simulink model "sampleModel248"  (R2021b)
settings: Solver=VariableStepAuto  StartTime=0.0  StopTime=10.0  RelTol=1e-3
undefined symbols (not defined in the file or in its folder): Newton, Raphson
libraries: simulink x15, slpidlib x4
settings Model: Creator=user  LastModifiedBy=user

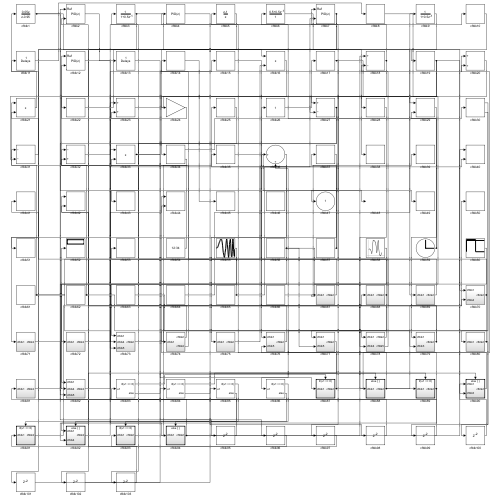
[thumbnail: Simulink's stored preview of the top-level diagram]
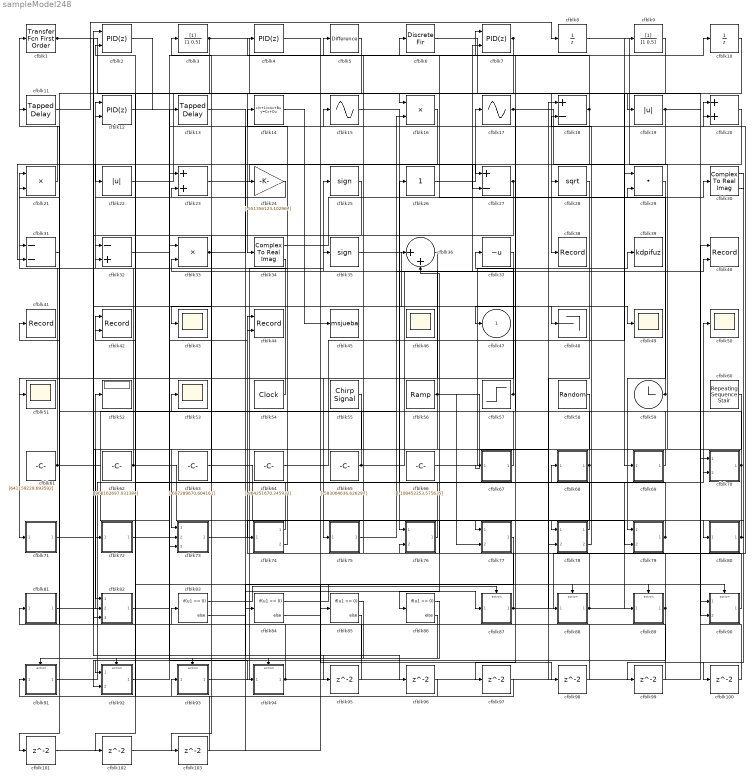
== system sampleModel248 ==
  cfblk1 : simulink/Discrete/Transfer Fcn First Order  PoleZ=0.95  ICPrevOutput=0.0  DoSatur=off
  cfblk10 : UnitDelay  HasFrameUpgradeWarning=on
  cfblk{95..103} (9 alike) : Delay  SampleTime=1
  cfblk11 : simulink/Discrete/Tapped Delay  vinit=0.0  samptime=-1  NumDelays=1  DelayOrder=Oldest  includeCurrent=off
  cfblk12 : slpidlib/PID Controller (2DOF)  Controller=PID  Form=Parallel  TimeDomain=Discrete-time  UseExternalTs=off  SampleTime=1  IntegratorMethod=Forward Euler  FilterMethod=Forward Euler  ControllerParametersSource=internal  P=1  I=1  D=0  UseFilter=on  N=100  b=1  c=1  TunerSelectOption=Transfer Function Based (PID Tuner App)  InitialConditionSource=internal  InitialConditionForIntegrator=0  InitialConditionForFilter=0  DifferentiatorICPrevScaledInput=0  ExternalReset=none  TrackingMode=off  Kt=1  LimitOutput=off  SatLimitsSource=internal  UpperSaturationLimit=inf  LowerSaturationLimit=-inf  LinearizeAsGain=off  AntiWindupMode=none  Kb=1  POutMin=[]  POutMax=[]  IOutMin=[]  IOutMax=[]  DOutMin=[]  DOutMax=[]  NOutMin=[]  NOutMax=[]  bOutMin=[]  bOutMax=[]  cOutMin=[]  cOutMax=[]  SumOutMin=[]  SumOutMax=[]  SaturationOutMin=[]  SaturationOutMax=[]  PParamMin=[]  PParamMax=[]  IParamMin=[]  IParamMax=[]  DParamMin=[]  DParamMax=[]  NParamMin=[]  NParamMax=[]  bParamMin=[]  bParamMax=[]  cParamMin=[]  cParamMax=[]  KbParamMin=[]  KbParamMax=[]  KtParamMin=[]  KtParamMax=[]  KbOutMin=[]  KbOutMax=[]  KtOutMin=[]  KtOutMax=[]  IntegratorOutMin=[]  IntegratorOutMax=[]  FilterOutMin=[]  FilterOutMax=[]  SumI1OutMin=[]  SumI1OutMax=[]  SumI2OutMin=[]  SumI2OutMax=[]  SumI3OutMin=[]  SumI3OutMax=[]  SumI4OutMin=[]  SumI4OutMax=[]  SumDOutMin=[]  SumDOutMax=[]  Sum1OutMin=[]  Sum1OutMax=[]  Sum2OutMin=[]  Sum2OutMax=[]  Sum3OutMin=[]  Sum3OutMax=[]  DifferentiatorOutMin=[]  DifferentiatorOutMax=[]  FilterDiffOutCoefMin=[]  FilterDiffOutCoefMax=[]  ReciprocalOutMin=[]  ReciprocalOutMax=[]  SumDenOutMin=[]  SumDenOutMax=[]  SumNumOutMin=[]  SumNumOutMax=[]  DivideOutMin=[]  DivideOutMax=[]  UdiffTsProdOutMin=[]  UdiffTsProdOutMax=[]  NTsProdOutMin=[]  NTsProdOutMax=[]  UintegralTsProdOutMin=[]  UintegralTsProdOutMax=[]  UngainTsProdOutMin=[]  UngainTsProdOutMax=[]  IntegratorContinuousStateAttributes=''  IntegratorStateMustResolveToSignalObject=off  IntegratorRTWStateStorageClass=Auto  FilterContinuousStateAttributes=''  FilterStateMustResolveToSignalObject=off  FilterRTWStateStorageClass=Auto  ParallelPVariant=InternalParameters  IdealPVariant=Disabled  IVariant=InternalParameters  DVariant=InternalParameters  bVariant=InternalParameters  cVariant=InternalParameters  IntegratorVariant=Discrete  SatVariant=Disabled  AWVariant=Passthrough  PCopyVariant=Disabled  TRVariant=Disabled  FdbkBlocksVariant=Forward  IdealPFdbkVariant=Disabled  SatFdbkVariant=Disabled  DerivativeFilterVariant=ForwardEulerFilter  NVariant=InternalParameters  NCopyVariant=Disabled  FilterICVariant=InternalICsFilter  IntegratorICVariant=InternalICs  ExternalResetVariant=Disabled  TRSumVariant=Passthrough  SumFdbkVariant=Disabled  SumVariant=Sum_PID  TsampFilterVariant=InternalTs  TsampNgainVariant=Passthrough  TsampIntegralVariant=Passthrough  ExternalSaturationOutDataTypeStr=Inherit: Same as second input
      settings: SourceProductBaseCode=SL
  cfblk13 : simulink/Discrete/Tapped Delay  vinit=0.0  samptime=-1  NumDelays=1  DelayOrder=Oldest  includeCurrent=off
  cfblk14 : DiscreteStateSpace
  cfblk15 : Sin  TimeSource=Use external signal  SampleTime=0
  cfblk16 : Product  Inputs=**
  cfblk17 : Sin  TimeSource=Use external signal  SampleTime=0
  cfblk18 : Sum  Inputs=+-
  cfblk19 : Abs
  cfblk2 : slpidlib/PID Controller (2DOF)  Controller=PID  Form=Parallel  TimeDomain=Discrete-time  UseExternalTs=off  SampleTime=1  IntegratorMethod=Forward Euler  FilterMethod=Forward Euler  ControllerParametersSource=internal  P=1  I=1  D=0  UseFilter=on  N=100  b=1  c=1  TunerSelectOption=Transfer Function Based (PID Tuner App)  InitialConditionSource=internal  InitialConditionForIntegrator=0  InitialConditionForFilter=0  DifferentiatorICPrevScaledInput=0  ExternalReset=none  TrackingMode=off  Kt=1  LimitOutput=off  SatLimitsSource=internal  UpperSaturationLimit=inf  LowerSaturationLimit=-inf  LinearizeAsGain=off  AntiWindupMode=none  Kb=1  POutMin=[]  POutMax=[]  IOutMin=[]  IOutMax=[]  DOutMin=[]  DOutMax=[]  NOutMin=[]  NOutMax=[]  bOutMin=[]  bOutMax=[]  cOutMin=[]  cOutMax=[]  SumOutMin=[]  SumOutMax=[]  SaturationOutMin=[]  SaturationOutMax=[]  PParamMin=[]  PParamMax=[]  IParamMin=[]  IParamMax=[]  DParamMin=[]  DParamMax=[]  NParamMin=[]  NParamMax=[]  bParamMin=[]  bParamMax=[]  cParamMin=[]  cParamMax=[]  KbParamMin=[]  KbParamMax=[]  KtParamMin=[]  KtParamMax=[]  KbOutMin=[]  KbOutMax=[]  KtOutMin=[]  KtOutMax=[]  IntegratorOutMin=[]  IntegratorOutMax=[]  FilterOutMin=[]  FilterOutMax=[]  SumI1OutMin=[]  SumI1OutMax=[]  SumI2OutMin=[]  SumI2OutMax=[]  SumI3OutMin=[]  SumI3OutMax=[]  SumI4OutMin=[]  SumI4OutMax=[]  SumDOutMin=[]  SumDOutMax=[]  Sum1OutMin=[]  Sum1OutMax=[]  Sum2OutMin=[]  Sum2OutMax=[]  Sum3OutMin=[]  Sum3OutMax=[]  DifferentiatorOutMin=[]  DifferentiatorOutMax=[]  FilterDiffOutCoefMin=[]  FilterDiffOutCoefMax=[]  ReciprocalOutMin=[]  ReciprocalOutMax=[]  SumDenOutMin=[]  SumDenOutMax=[]  SumNumOutMin=[]  SumNumOutMax=[]  DivideOutMin=[]  DivideOutMax=[]  UdiffTsProdOutMin=[]  UdiffTsProdOutMax=[]  NTsProdOutMin=[]  NTsProdOutMax=[]  UintegralTsProdOutMin=[]  UintegralTsProdOutMax=[]  UngainTsProdOutMin=[]  UngainTsProdOutMax=[]  IntegratorContinuousStateAttributes=''  IntegratorStateMustResolveToSignalObject=off  IntegratorRTWStateStorageClass=Auto  FilterContinuousStateAttributes=''  FilterStateMustResolveToSignalObject=off  FilterRTWStateStorageClass=Auto  ParallelPVariant=InternalParameters  IdealPVariant=Disabled  IVariant=InternalParameters  DVariant=InternalParameters  bVariant=InternalParameters  cVariant=InternalParameters  IntegratorVariant=Discrete  SatVariant=Disabled  AWVariant=Passthrough  PCopyVariant=Disabled  TRVariant=Disabled  FdbkBlocksVariant=Forward  IdealPFdbkVariant=Disabled  SatFdbkVariant=Disabled  DerivativeFilterVariant=ForwardEulerFilter  NVariant=InternalParameters  NCopyVariant=Disabled  FilterICVariant=InternalICsFilter  IntegratorICVariant=InternalICs  ExternalResetVariant=Disabled  TRSumVariant=Passthrough  SumFdbkVariant=Disabled  SumVariant=Sum_PID  TsampFilterVariant=InternalTs  TsampNgainVariant=Passthrough  TsampIntegralVariant=Passthrough  ExternalSaturationOutDataTypeStr=Inherit: Same as second input
      settings: SourceProductBaseCode=SL
  cfblk20 : Sum
  cfblk21 : Product
  cfblk22 : Abs
  cfblk23 : Sum
  cfblk24 : Gain  Gain=[-551356123.102967]
  cfblk25 : Signum
  cfblk26 : simulink/Math Operations/Slider Gain  gain=1  low=0  high=2
  cfblk27 : Sum  Inputs=+-
  cfblk28 : Sqrt  SaturateOnIntegerOverflow=on
  cfblk29 : DotProduct  InputSameDT=on  OutDataTypeStr=Inherit: Inherit via internal rule
  cfblk3 : DiscreteFilter  SampleTime=1
  cfblk30 : ComplexToRealImag
  cfblk31 : Sum  Inputs=--
  cfblk32 : Sum  Inputs=-+
  cfblk33 : Product  Inputs=**
  cfblk34 : ComplexToRealImag
  cfblk35 : Signum
  cfblk36 : Sum  Inputs=|++
  cfblk37 : UnaryMinus
  cfblk38 : Record  FileSettingsInternal="{\"entries\":[{\"content\":{\"excelSettings\":{\"content\":{},\"type\":\"Streamout.ExcelSettings\"}},\"type\":\"Streamout.FileSettingStorage\",\"uuid\":\"4657b973-2eff-446c-9fb0-9f6287b31807\"}],\"packageUris\":[\"http://schema.mathworks.com/mf0/streamout_blocks/R2020a\"],\"version\":\"1.0\"}"  SignalsInternal="{\"entries\":[{\"content\":{\"signals\":[{\"content\":{\"blockPath\":[\"sampleModel248/cfblk38\"],\"channel\":[],\"dimensions\":[1],\"domain\":\"sampleModel248/cfblk38\",\"lineColor\":\"#ff13a6\",\"plots\":[1],\"port\":1,\"sid\":[\"\"],\"signalID\":9988,\"signalName\":\"cfblk1\"},\"type\":\"RecordBlkView.Signal\",\"uuid\":\"57bce957-2fdd-423c-8d0d-79339184f327\"}]},\"type\":\"RecordBlkView.InputSignals\",\"uuid\":\"285c4055-8f1f-46df-a613-131e11705366\"}],\"packageUris\":[\"http://schema.mathworks.com/mf0/streamout_blocks/R2020a\"],\"version\":\"1.0\"}"  VisualizationBindings="{\"sparklinesplugin\":{\"info\":[{\"bindingParametersList\":[],\"subplotID\":1}]}}"
  cfblk39 : ToWorkspace  VariableName=kdpifuz  SaveFormat=Timeseries  SampleTime=-1
  cfblk4 : slpidlib/PID Controller  Controller=PID  Form=Parallel  TimeDomain=Discrete-time  UseExternalTs=off  SampleTime=1  IntegratorMethod=Forward Euler  FilterMethod=Forward Euler  ControllerParametersSource=internal  P=1  I=1  D=0  UseFilter=on  N=100  TunerSelectOption=Transfer Function Based (PID Tuner App)  InitialConditionSource=internal  InitialConditionForIntegrator=0  InitialConditionForFilter=0  DifferentiatorICPrevScaledInput=0  ExternalReset=none  TrackingMode=off  Kt=1  LimitOutput=off  SatLimitsSource=internal  UpperSaturationLimit=inf  LowerSaturationLimit=-inf  LinearizeAsGain=off  AntiWindupMode=none  Kb=1  POutMin=[]  POutMax=[]  IOutMin=[]  IOutMax=[]  DOutMin=[]  DOutMax=[]  NOutMin=[]  NOutMax=[]  SumOutMin=[]  SumOutMax=[]  SaturationOutMin=[]  SaturationOutMax=[]  PParamMin=[]  PParamMax=[]  IParamMin=[]  IParamMax=[]  DParamMin=[]  DParamMax=[]  NParamMin=[]  NParamMax=[]  KbParamMin=[]  KbParamMax=[]  KtParamMin=[]  KtParamMax=[]  KbOutMin=[]  KbOutMax=[]  KtOutMin=[]  KtOutMax=[]  IntegratorOutMin=[]  IntegratorOutMax=[]  FilterOutMin=[]  FilterOutMax=[]  SumI1OutMin=[]  SumI1OutMax=[]  SumI2OutMin=[]  SumI2OutMax=[]  SumI3OutMin=[]  SumI3OutMax=[]  SumI4OutMin=[]  SumI4OutMax=[]  SumDOutMin=[]  SumDOutMax=[]  DifferentiatorOutMin=[]  DifferentiatorOutMax=[]  FilterDiffOutCoefMin=[]  FilterDiffOutCoefMax=[]  ReciprocalOutMin=[]  ReciprocalOutMax=[]  SumDenOutMin=[]  SumDenOutMax=[]  SumNumOutMin=[]  SumNumOutMax=[]  DivideOutMin=[]  DivideOutMax=[]  UdiffTsProdOutMin=[]  UdiffTsProdOutMax=[]  NTsProdOutMin=[]  NTsProdOutMax=[]  UintegralTsProdOutMin=[]  UintegralTsProdOutMax=[]  UngainTsProdOutMin=[]  UngainTsProdOutMax=[]  IntegratorContinuousStateAttributes=''  IntegratorStateMustResolveToSignalObject=off  IntegratorRTWStateStorageClass=Auto  FilterContinuousStateAttributes=''  FilterStateMustResolveToSignalObject=off  FilterRTWStateStorageClass=Auto  ParallelPVariant=InternalParameters  IdealPVariant=Disabled  IVariant=InternalParameters  DVariant=InternalParameters  IntegratorVariant=Discrete  SatVariant=Disabled  AWVariant=Passthrough  PCopyVariant=Disabled  TRVariant=Disabled  FdbkBlocksVariant=Forward  IdealPFdbkVariant=Disabled  SatFdbkVariant=Disabled  DerivativeFilterVariant=ForwardEulerFilter  NVariant=InternalParameters  NCopyVariant=Disabled  FilterICVariant=InternalICsFilter  IntegratorICVariant=InternalICs  ExternalResetVariant=Disabled  TRSumVariant=Passthrough  SumFdbkVariant=Disabled  SumVariant=Sum_PID  TsampFilterVariant=InternalTs  TsampNgainVariant=Passthrough  TsampIntegralVariant=Passthrough  ExternalSaturationOutDataTypeStr=Inherit: Same as second input
  cfblk40 : Record  FileSettingsInternal="{\"entries\":[{\"content\":{\"excelSettings\":{\"content\":{},\"type\":\"Streamout.ExcelSettings\"}},\"type\":\"Streamout.FileSettingStorage\",\"uuid\":\"e8e254c2-0b66-4196-82d5-06a13f5ebabd\"}],\"packageUris\":[\"http://schema.mathworks.com/mf0/streamout_blocks/R2020a\"],\"version\":\"1.0\"}"  Layout=[1 1]  SignalsInternal="{\"entries\":[{\"content\":{\"signals\":[{\"content\":{\"blockPath\":[\"sampleModel248/cfblk40\"],\"channel\":[],\"dimensions\":[1],\"domain\":\"sampleModel248/cfblk40\",\"lineColor\":\"#a2142f\",\"plots\":[1],\"port\":1,\"sid\":[\"\"],\"signalID\":9992,\"signalName\":\"cfblk94\"},\"type\":\"RecordBlkView.Signal\",\"uuid\":\"96483212-cd48-427b-a849-b49e468cae1c\"},{\"content\":{\"blockPath\":[\"sampleModel248/cfblk40\"],\"channel\":[],\"dimensions\":[1],\"domain\":\"sampleModel248/cfblk40\",\"lineColor\":\"#139fff\",\"plots\":[1],\"port\":2,\"sid\":[\"\"],\"signalID\":9996,\"signalName\":\"cfblk75\"},\"type\":\"RecordBlkView.Signal\",\"uuid\":\"ecaeb14c-769c-40d5-b804-4b1f23d1b747\"}]},\"type\":\"RecordBlkView.InputSignals\",\"uuid\":\"bcef0295-5273-4388-9474-6ff76888c008\"}],\"packageUris\":[\"http://schema.mathworks.com/mf0/streamout_blocks/R2020a\"],\"version\":\"1.0\"}"  VisualizationBindings="{\"xyplotplugin\":{\"info\":[{\"series\":[{\"bindingParametersList\":[{\"parameter\":\"X-Axis\",\"signalID\":9992,\"signalName\":\"cfblk94\"},{\"parameter\":\"Y-Axis\",\"signalID\":9996,\"signalName\":\"cfblk75\"}],\"seriesID\":20823}],\"subplotID\":1}]}}"  CompatibilityTag=XY
  cfblk41 : Record  FileSettingsInternal="{\"entries\":[{\"content\":{\"excelSettings\":{\"content\":{},\"type\":\"Streamout.ExcelSettings\"}},\"type\":\"Streamout.FileSettingStorage\",\"uuid\":\"af2688e8-db05-4c26-a761-651d88233be8\"}],\"packageUris\":[\"http://schema.mathworks.com/mf0/streamout_blocks/R2020a\"],\"version\":\"1.0\"}"  SignalsInternal="{\"entries\":[{\"content\":{\"signals\":[{\"content\":{\"blockPath\":[\"sampleModel248/cfblk41\"],\"channel\":[],\"dimensions\":[1],\"domain\":\"sampleModel248/cfblk41\",\"lineColor\":\"#0072bd\",\"plots\":[1],\"port\":1,\"sid\":[\"\"],\"signalID\":10000,\"signalName\":\"cfblk94\"},\"type\":\"RecordBlkView.Signal\",\"uuid\":\"c2de7e0d-ba0f-46c5-868c-2fe38e3ac21e\"}]},\"type\":\"RecordBlkView.InputSignals\",\"uuid\":\"3469a304-3501-4b95-a551-717c17ac85cc\"}],\"packageUris\":[\"http://schema.mathworks.com/mf0/streamout_blocks/R2020a\"],\"version\":\"1.0\"}"  VisualizationBindings="{\"sparklinesplugin\":{\"info\":[{\"bindingParametersList\":[],\"subplotID\":1}]}}"
  cfblk42 : Record  FileSettingsInternal="{\"entries\":[{\"content\":{\"excelSettings\":{\"content\":{},\"type\":\"Streamout.ExcelSettings\"}},\"type\":\"Streamout.FileSettingStorage\",\"uuid\":\"8a6774b2-f76e-4be7-b4b1-672b2e9fdf31\"}],\"packageUris\":[\"http://schema.mathworks.com/mf0/streamout_blocks/R2020a\"],\"version\":\"1.0\"}"  Layout=[1 1]  SignalsInternal="{\"entries\":[{\"content\":{\"signals\":[{\"content\":{\"blockPath\":[\"sampleModel248/cfblk42\"],\"channel\":[],\"dimensions\":[1],\"domain\":\"sampleModel248/cfblk42\",\"lineColor\":\"#a2142f\",\"plots\":[1],\"port\":1,\"sid\":[\"\"],\"signalID\":10004,\"signalName\":\"cfblk79\"},\"type\":\"RecordBlkView.Signal\",\"uuid\":\"6845512b-980a-4326-b86a-4d7e02a87132\"},{\"content\":{\"blockPath\":[\"sampleModel248/cfblk42\"],\"channel\":[],\"dimensions\":[1],\"domain\":\"sampleModel248/cfblk42\",\"lineColor\":\"#139fff\",\"plots\":[1],\"port\":2,\"sid\":[\"\"],\"signalID\":10008,\"signalName\":\"cfblk74:1\"},\"type\":\"RecordBlkView.Signal\",\"uuid\":\"88b51775-9405-4252-8d6c-4fb987ba6e22\"}]},\"type\":\"RecordBlkView.InputSignals\",\"uuid\":\"851e467b-af1b-40f0-a187-e79c8d2d79f2\"}],\"packageUris\":[\"http://schema.mathworks.com/mf0/streamout_blocks/R2020a\"],\"version\":\"1.0\"}"  VisualizationBindings="{\"xyplotplugin\":{\"info\":[{\"series\":[{\"bindingParametersList\":[{\"parameter\":\"X-Axis\",\"signalID\":10004,\"signalName\":\"cfblk79\"},{\"parameter\":\"Y-Axis\",\"signalID\":10008,\"signalName\":\"cfblk74:1\"}],\"seriesID\":11787}],\"subplotID\":1}]}}"  CompatibilityTag=XY
  cfblk{43,46,49..51,53} (6 alike) : Scope
      cfblk46 settings: Floating=on
  cfblk44 : Record  FileSettingsInternal="{\"entries\":[{\"content\":{\"excelSettings\":{\"content\":{},\"type\":\"Streamout.ExcelSettings\"}},\"type\":\"Streamout.FileSettingStorage\",\"uuid\":\"38156eca-3516-4139-b23b-3a3a441e8744\"}],\"packageUris\":[\"http://schema.mathworks.com/mf0/streamout_blocks/R2020a\"],\"version\":\"1.0\"}"  Layout=[1 1]  SignalsInternal="{\"entries\":[{\"content\":{\"signals\":[{\"content\":{\"blockPath\":[\"sampleModel248/cfblk44\"],\"channel\":[],\"dimensions\":[1],\"domain\":\"sampleModel248/cfblk44\",\"lineColor\":\"#a2142f\",\"plots\":[1],\"port\":1,\"sid\":[\"\"],\"signalID\":10012,\"signalName\":\"cfblk72\"},\"type\":\"RecordBlkView.Signal\",\"uuid\":\"63087910-4408-4e77-b969-9ff7fd655d93\"},{\"content\":{\"blockPath\":[\"sampleModel248/cfblk44\"],\"channel\":[],\"dimensions\":[1],\"domain\":\"sampleModel248/cfblk44\",\"lineColor\":\"#139fff\",\"plots\":[1],\"port\":2,\"sid\":[\"\"],\"signalID\":10016,\"signalName\":\"cfblk88\"},\"type\":\"RecordBlkView.Signal\",\"uuid\":\"23e4db46-6528-4736-b7aa-4516a92a3fc2\"}]},\"type\":\"RecordBlkView.InputSignals\",\"uuid\":\"3ac9fc90-d2c7-4ec6-9b36-f304a41b0667\"}],\"packageUris\":[\"http://schema.mathworks.com/mf0/streamout_blocks/R2020a\"],\"version\":\"1.0\"}"  VisualizationBindings="{\"xyplotplugin\":{\"info\":[{\"series\":[{\"bindingParametersList\":[{\"parameter\":\"X-Axis\",\"signalID\":10012,\"signalName\":\"cfblk72\"},{\"parameter\":\"Y-Axis\",\"signalID\":10016,\"signalName\":\"cfblk88\"}],\"seriesID\":2509}],\"subplotID\":1}]}}"  CompatibilityTag=XY
  cfblk45 : ToWorkspace  VariableName=msjueba  SaveFormat=Timeseries  SampleTime=-1
  cfblk48 : Terminator
  cfblk5 : simulink/Discrete/Difference  ICPrevInput=0.0  OutMin=[]  OutMax=[]  OutDataTypeStr=Inherit: Inherit via back propagation  OutDataType=fixdt(1, 16)  OutScaling=2^-10  DoSatur=off
  cfblk52 : Display
  cfblk54 : DigitalClock
  cfblk55 : simulink/Sources/Chirp Signal  f1=[-842753396.758017]  T=[-513335603.645566]  f2=[469948596.310071]
  cfblk56 : simulink/Sources/Ramp  slope=[9429.766515]  start=[8.370779]  InitialOutput=[865254.958316]
  cfblk57 : Step  Time=[16.000000]  Before=[-143517300.049279]  After=[-931102993.067420]  SampleTime=0
  cfblk58 : RandomNumber  Mean=[-94668.812699]  Variance=[59598.162771]  Seed=[243885684.000000]  SampleTime=0.1
  cfblk59 : Clock
  cfblk6 : DiscreteFir  SampleTime=1
  cfblk60 : simulink/Sources/Repeating Sequence Stair  OutValues=[94042115.730046, -975852631.296547]  tsamp=-1  OutMin=[]  OutMax=[]  OutDataTypeStr=double  OutputDataTypeScalingMode=double  OutDataType=fixdt(0,8)  ConRadixGroup=Best Precision: Vector-wise  OutScaling=2^-12
  cfblk61 : Constant  Value=[641159229.693592]  SampleTime=1
  cfblk62 : Constant  Value=[868162697.031384]  SampleTime=1
  cfblk63 : Constant  Value=[-697289670.604161]  SampleTime=1
  cfblk64 : Constant  Value=[-864251670.245932]  SampleTime=1
  cfblk65 : Constant  Value=[-583064636.626297]  SampleTime=1
  cfblk66 : Constant  Value=[-108452253.575635]  SampleTime=1
  cfblk67 : Subsystem
  cfblk68 : Subsystem
  cfblk69 : Subsystem
  cfblk7 : slpidlib/PID Controller (2DOF)  Controller=PID  Form=Parallel  TimeDomain=Discrete-time  UseExternalTs=off  SampleTime=1  IntegratorMethod=Forward Euler  FilterMethod=Forward Euler  ControllerParametersSource=internal  P=1  I=1  D=0  UseFilter=on  N=100  b=1  c=1  TunerSelectOption=Transfer Function Based (PID Tuner App)  InitialConditionSource=internal  InitialConditionForIntegrator=0  InitialConditionForFilter=0  DifferentiatorICPrevScaledInput=0  ExternalReset=none  TrackingMode=off  Kt=1  LimitOutput=off  SatLimitsSource=internal  UpperSaturationLimit=inf  LowerSaturationLimit=-inf  LinearizeAsGain=off  AntiWindupMode=none  Kb=1  POutMin=[]  POutMax=[]  IOutMin=[]  IOutMax=[]  DOutMin=[]  DOutMax=[]  NOutMin=[]  NOutMax=[]  bOutMin=[]  bOutMax=[]  cOutMin=[]  cOutMax=[]  SumOutMin=[]  SumOutMax=[]  SaturationOutMin=[]  SaturationOutMax=[]  PParamMin=[]  PParamMax=[]  IParamMin=[]  IParamMax=[]  DParamMin=[]  DParamMax=[]  NParamMin=[]  NParamMax=[]  bParamMin=[]  bParamMax=[]  cParamMin=[]  cParamMax=[]  KbParamMin=[]  KbParamMax=[]  KtParamMin=[]  KtParamMax=[]  KbOutMin=[]  KbOutMax=[]  KtOutMin=[]  KtOutMax=[]  IntegratorOutMin=[]  IntegratorOutMax=[]  FilterOutMin=[]  FilterOutMax=[]  SumI1OutMin=[]  SumI1OutMax=[]  SumI2OutMin=[]  SumI2OutMax=[]  SumI3OutMin=[]  SumI3OutMax=[]  SumI4OutMin=[]  SumI4OutMax=[]  SumDOutMin=[]  SumDOutMax=[]  Sum1OutMin=[]  Sum1OutMax=[]  Sum2OutMin=[]  Sum2OutMax=[]  Sum3OutMin=[]  Sum3OutMax=[]  DifferentiatorOutMin=[]  DifferentiatorOutMax=[]  FilterDiffOutCoefMin=[]  FilterDiffOutCoefMax=[]  ReciprocalOutMin=[]  ReciprocalOutMax=[]  SumDenOutMin=[]  SumDenOutMax=[]  SumNumOutMin=[]  SumNumOutMax=[]  DivideOutMin=[]  DivideOutMax=[]  UdiffTsProdOutMin=[]  UdiffTsProdOutMax=[]  NTsProdOutMin=[]  NTsProdOutMax=[]  UintegralTsProdOutMin=[]  UintegralTsProdOutMax=[]  UngainTsProdOutMin=[]  UngainTsProdOutMax=[]  IntegratorContinuousStateAttributes=''  IntegratorStateMustResolveToSignalObject=off  IntegratorRTWStateStorageClass=Auto  FilterContinuousStateAttributes=''  FilterStateMustResolveToSignalObject=off  FilterRTWStateStorageClass=Auto  ParallelPVariant=InternalParameters  IdealPVariant=Disabled  IVariant=InternalParameters  DVariant=InternalParameters  bVariant=InternalParameters  cVariant=InternalParameters  IntegratorVariant=Discrete  SatVariant=Disabled  AWVariant=Passthrough  PCopyVariant=Disabled  TRVariant=Disabled  FdbkBlocksVariant=Forward  IdealPFdbkVariant=Disabled  SatFdbkVariant=Disabled  DerivativeFilterVariant=ForwardEulerFilter  NVariant=InternalParameters  NCopyVariant=Disabled  FilterICVariant=InternalICsFilter  IntegratorICVariant=InternalICs  ExternalResetVariant=Disabled  TRSumVariant=Passthrough  SumFdbkVariant=Disabled  SumVariant=Sum_PID  TsampFilterVariant=InternalTs  TsampNgainVariant=Passthrough  TsampIntegralVariant=Passthrough  ExternalSaturationOutDataTypeStr=Inherit: Same as second input
      settings: SourceProductBaseCode=SL
  cfblk70 : Subsystem
  cfblk71 : Subsystem
  cfblk72 : Subsystem
  cfblk73 : Subsystem
  cfblk74 : Subsystem
  cfblk75 : Subsystem
  cfblk76 : Subsystem
  cfblk77 : Subsystem
  cfblk78 : Subsystem
  cfblk79 : Subsystem
  cfblk8 : UnitDelay  HasFrameUpgradeWarning=on
  cfblk80 : Subsystem
  cfblk81 : Subsystem
  cfblk82 : Subsystem
  cfblk{83..86} (4 alike) : If  IfExpression=u1 >= 0  SampleTime=1
  cfblk87 : Subsystem  TreatAsAtomicUnit=on
  cfblk88 : Subsystem  TreatAsAtomicUnit=on
  cfblk89 : Subsystem  TreatAsAtomicUnit=on
  cfblk9 : DiscreteFilter  SampleTime=1
  cfblk90 : Subsystem  TreatAsAtomicUnit=on
  cfblk91 : Subsystem  TreatAsAtomicUnit=on
  cfblk92 : Subsystem  TreatAsAtomicUnit=on
  cfblk93 : Subsystem  TreatAsAtomicUnit=on
  cfblk94 : Subsystem  TreatAsAtomicUnit=on
  cfblk47 : Outport
  wires:
  cfblk55/1 -> cfblk73/1(cfblk1)
  cfblk14/1 -> cfblk45/1
  cfblk22/1 -> cfblk16/1
  cfblk93/1(cfblk2) -> cfblk50/1
  cfblk66/1 -> cfblk39/1
  cfblk24/1 -> cfblk12/1
  cfblk2/1 -> cfblk13/1
  cfblk11/1 -> cfblk8/1
  cfblk59/1 -> cfblk6/1, cfblk29/2
  cfblk8/1 -> cfblk67/1(cfblk1)
  cfblk15/1 -> cfblk76/1(cfblk1)
  cfblk68/1(cfblk2) -> cfblk86/1, cfblk23/2
  cfblk63/1 -> cfblk78/1(cfblk1)
  cfblk37/1 -> cfblk75/1(cfblk1)
  cfblk61/1 -> cfblk21/1, cfblk73/2(cfblk4), cfblk16/2
  cfblk31/1 -> cfblk1/1
  cfblk26/1 -> cfblk17/1
  cfblk33/1 -> cfblk20/2, cfblk96/1
  cfblk81/1(cfblk2) -> cfblk52/1
  cfblk36/1 -> cfblk71/1(cfblk1)
  cfblk54/1 -> cfblk12/2
  cfblk69/1(cfblk2) -> cfblk7/1
  cfblk9/1 -> cfblk19/1
  cfblk6/1 -> cfblk70/1(cfblk1)
  cfblk92/1(cfblk2) -> cfblk33/1
  cfblk65/1 -> cfblk7/2, cfblk21/2
  cfblk10/1 -> cfblk34/1
  cfblk70/1(cfblk2) -> cfblk14/1, cfblk74/1(cfblk1)
  cfblk91/1(cfblk2) -> cfblk68/1(cfblk1)
  cfblk30/2 -> cfblk80/1(cfblk1)
  cfblk13/1 -> cfblk87/1(cfblk1)
  cfblk35/1 -> cfblk49/1
  cfblk21/1 -> cfblk11/1
  cfblk34/1 -> cfblk30/1
  cfblk87/1(cfblk2) -> cfblk20/1, cfblk36/2
  cfblk23/1 -> cfblk27/1
  cfblk29/1 -> cfblk79/1(cfblk1)
  cfblk80/1(cfblk2) -> cfblk77/1(cfblk1), cfblk100/1
  cfblk1/1 -> cfblk38/1, cfblk48/1
  cfblk34/2 -> cfblk31/1
  cfblk18/1 -> cfblk4/1, cfblk97/1
  cfblk58/1 -> cfblk82/1(cfblk1)
  cfblk56/1 -> cfblk72/1(cfblk1), cfblk35/1, cfblk77/2(cfblk5), cfblk88/1(cfblk1)
  cfblk73/1(cfblk2) -> cfblk25/1
  cfblk57/1 -> cfblk33/2, cfblk37/1
  cfblk28/1 -> cfblk78/2(cfblk4)
  cfblk82/1(cfblk2) -> cfblk10/1
  cfblk76/1(cfblk2) -> cfblk3/1
  cfblk88/1(cfblk2) -> cfblk89/1(cfblk1), cfblk44/2, cfblk70/2(cfblk4)
  cfblk16/1 -> cfblk24/1
  cfblk17/1 -> cfblk47/1, cfblk69/1(cfblk1)
  cfblk72/1(cfblk2) -> cfblk44/1
  cfblk19/1 -> cfblk90/2(cfblk3), cfblk27/2, cfblk28/1, cfblk73/3(cfblk5)
  cfblk12/1 -> cfblk94/1(cfblk1)
  cfblk25/1 -> cfblk43/1
  cfblk94/1(cfblk2) -> cfblk40/1, cfblk41/1, cfblk18/1
  cfblk90/1(cfblk2) -> cfblk5/1
  cfblk32/1 -> cfblk15/1
  cfblk75/1(cfblk2) -> cfblk40/2
  cfblk79/1(cfblk2) -> cfblk42/1, cfblk18/2
  cfblk60/1 -> cfblk82/2(cfblk4)
  cfblk64/1 -> cfblk9/1
  cfblk74/1(cfblk2) -> cfblk42/2
  cfblk20/1 -> cfblk31/2
  cfblk89/1(cfblk2) -> cfblk81/1(cfblk1), cfblk92/2(cfblk4), cfblk76/2(cfblk5)
  cfblk3/1 -> cfblk51/1, cfblk29/1
  cfblk27/1 -> cfblk82/3(cfblk5), cfblk103/1
  cfblk62/1 -> cfblk79/2(cfblk3), cfblk32/2
  cfblk74/2(cfblk4) -> cfblk32/1
  cfblk7/1 -> cfblk92/1(cfblk1), cfblk22/1
  cfblk67/1(cfblk2) -> cfblk26/1
  cfblk78/1(cfblk2) -> cfblk36/1
  cfblk78/2(cfblk5) -> cfblk53/1
  cfblk83/1 -> cfblk87/Action
  cfblk83/2 -> cfblk88/Action
  cfblk84/1 -> cfblk89/Action
  cfblk84/2 -> cfblk90/Action
  cfblk85/1 -> cfblk91/Action
  cfblk85/2 -> cfblk92/Action
  cfblk86/1 -> cfblk93/Action
  cfblk86/2 -> cfblk94/Action
  cfblk71/1(cfblk2) -> cfblk95/1
  cfblk95/1 -> cfblk83/1
  cfblk96/1 -> cfblk91/1(cfblk1)
  cfblk97/1 -> cfblk93/1(cfblk1)
  cfblk4/1 -> cfblk98/1
  cfblk98/1 -> cfblk2/1
  cfblk30/1 -> cfblk99/1
  cfblk99/1 -> cfblk23/1
  cfblk100/1 -> cfblk90/1(cfblk1)
  cfblk5/1 -> cfblk101/1
  cfblk101/1 -> cfblk84/1
  cfblk77/1(cfblk2) -> cfblk102/1
  cfblk102/1 -> cfblk85/1
  cfblk103/1 -> cfblk2/2

== system sampleModel248/cfblk67 ==
  cfblk1 : Inport
  cfblk3 : Sum  Inputs=+-
  cfblk2 : Outport
  wires:
  cfblk1/1 -> cfblk3/1, cfblk3/2
  cfblk3/1 -> cfblk2/1

== system sampleModel248/cfblk68 ==
  cfblk1 : Inport
  cfblk3 : Gain  Gain=[785918242.816621]
  cfblk2 : Outport
  wires:
  cfblk1/1 -> cfblk2/1, cfblk3/1

== system sampleModel248/cfblk69 ==
  cfblk1 : Inport
  cfblk3 : Sqrt  Operator=rSqrt  AlgorithmType=Newton-Raphson  SaturateOnIntegerOverflow=on
  cfblk2 : Outport
  wires:
  cfblk1/1 -> cfblk3/1
  cfblk3/1 -> cfblk2/1

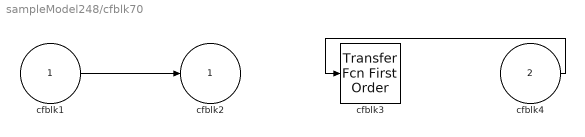
== system sampleModel248/cfblk70 ==
  cfblk1 : Inport
  cfblk4 : Inport  Port=2
  cfblk3 : simulink/Discrete/Transfer Fcn First Order  PoleZ=0.95  ICPrevOutput=0.0  DoSatur=off
  cfblk2 : Outport
  wires:
  cfblk4/1 -> cfblk3/1
  cfblk1/1 -> cfblk2/1

== system sampleModel248/cfblk71 ==
  cfblk1 : Inport
  cfblk3 : Product  Inputs=**
  cfblk2 : Outport
  wires:
  cfblk1/1 -> cfblk3/1, cfblk3/2
  cfblk3/1 -> cfblk2/1

== system sampleModel248/cfblk72 ==
  cfblk1 : Inport
  cfblk3 : simulink/Math Operations/MinMax Running Resettable  Function=min  vinit=0.0
  cfblk2 : Outport
  wires:
  cfblk1/1 -> cfblk2/1, cfblk3/1, cfblk3/2

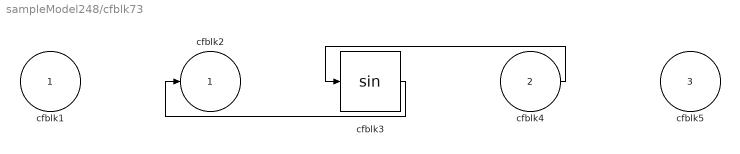
== system sampleModel248/cfblk73 ==
  cfblk1 : Inport
  cfblk4 : Inport  Port=2
  cfblk5 : Inport  Port=3
  cfblk3 : Trigonometry
  cfblk2 : Outport
  wires:
  cfblk4/1 -> cfblk3/1
  cfblk3/1 -> cfblk2/1

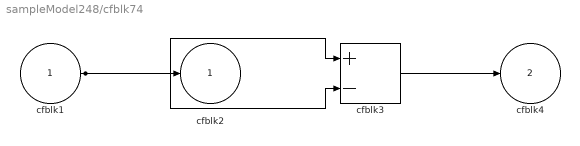
== system sampleModel248/cfblk74 ==
  cfblk1 : Inport
  cfblk3 : Sum  Inputs=+-
  cfblk2 : Outport
  cfblk4 : Outport  Port=2
  wires:
  cfblk1/1 -> cfblk3/1, cfblk3/2, cfblk2/1
  cfblk3/1 -> cfblk4/1

== system sampleModel248/cfblk75 ==
  cfblk1 : Inport
  cfblk3 : Sqrt  Operator=rSqrt  AlgorithmType=Newton-Raphson  SaturateOnIntegerOverflow=on
  cfblk4 : Constant  Value=[370546826.301811]  SampleTime=1
  cfblk2 : Outport
  wires:
  cfblk4/1 -> cfblk3/1
  cfblk3/1 -> cfblk2/1

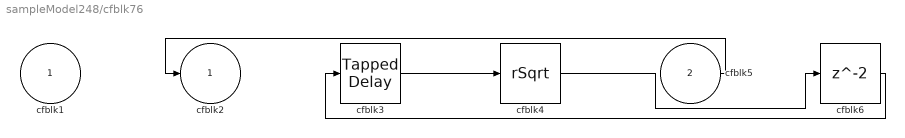
== system sampleModel248/cfblk76 ==
  cfblk1 : Inport
  cfblk5 : Inport  Port=2
  cfblk3 : simulink/Discrete/Tapped Delay  vinit=0.0  samptime=-1  NumDelays=1  DelayOrder=Oldest  includeCurrent=off
  cfblk4 : Sqrt  Operator=rSqrt  AlgorithmType=Newton-Raphson  SaturateOnIntegerOverflow=on
  cfblk6 : Delay  SampleTime=1
  cfblk2 : Outport
  wires:
  cfblk5/1 -> cfblk2/1
  cfblk3/1 -> cfblk4/1
  cfblk4/1 -> cfblk6/1
  cfblk6/1 -> cfblk3/1

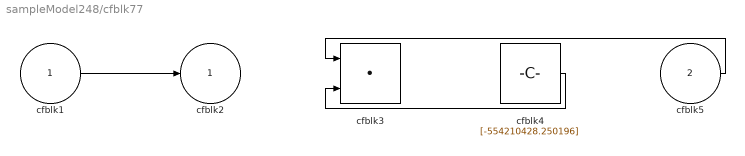
== system sampleModel248/cfblk77 ==
  cfblk1 : Inport
  cfblk5 : Inport  Port=2
  cfblk3 : DotProduct  InputSameDT=on  OutDataTypeStr=Inherit: Inherit via internal rule
  cfblk4 : Constant  Value=[-554210428.250196]  SampleTime=1
  cfblk2 : Outport
  wires:
  cfblk1/1 -> cfblk2/1
  cfblk5/1 -> cfblk3/1
  cfblk4/1 -> cfblk3/2

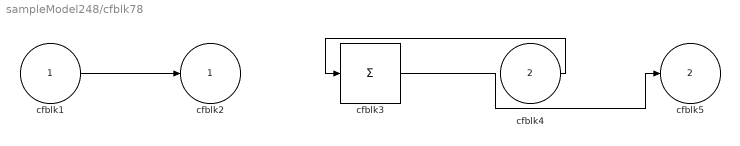
== system sampleModel248/cfblk78 ==
  cfblk1 : Inport
  cfblk4 : Inport  Port=2
  cfblk3 : Sum  Inputs=+
  cfblk2 : Outport
  cfblk5 : Outport  Port=2
  wires:
  cfblk4/1 -> cfblk3/1
  cfblk3/1 -> cfblk5/1
  cfblk1/1 -> cfblk2/1

== system sampleModel248/cfblk79 ==
  cfblk1 : Inport
  cfblk3 : Inport  Port=2
  cfblk2 : Outport
  wires:
  cfblk1/1 -> cfblk2/1

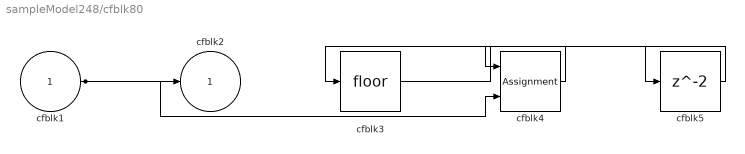
== system sampleModel248/cfblk80 ==
  cfblk1 : Inport
  cfblk3 : Rounding
  cfblk4 : Assignment  DiagnosticForDimensions=Warning  IndexOptions=Index vector (dialog)  Indices=1  OutputSizes=1
  cfblk5 : Delay  SampleTime=1
  cfblk2 : Outport
  wires:
  cfblk4/1 -> cfblk3/1
  cfblk1/1 -> cfblk2/1, cfblk4/2
  cfblk3/1 -> cfblk5/1
  cfblk5/1 -> cfblk4/1

== system sampleModel248/cfblk81 ==
  cfblk1 : Inport
  cfblk3 : simulink/Discrete/Transfer Fcn Lead or Lag  PoleZ=0.95  ZeroZ=0.75  ICPrevOutput=0.0  ICPrevInput=0.0  DoSatur=off
      settings: SourceProductBaseCode=SL
  cfblk2 : Outport
  wires:
  cfblk1/1 -> cfblk3/1
  cfblk3/1 -> cfblk2/1

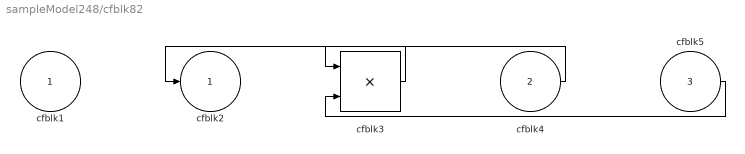
== system sampleModel248/cfblk82 ==
  cfblk1 : Inport
  cfblk4 : Inport  Port=2
  cfblk5 : Inport  Port=3
  cfblk3 : Product  Inputs=**
  cfblk2 : Outport
  wires:
  cfblk4/1 -> cfblk3/1
  cfblk5/1 -> cfblk3/2
  cfblk3/1 -> cfblk2/1

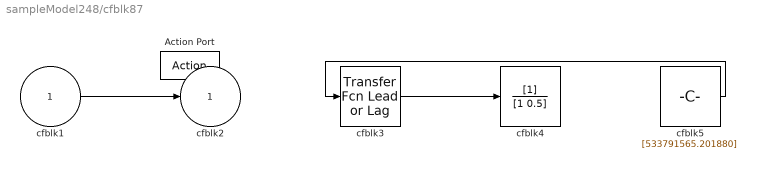
== system sampleModel248/cfblk87 ==
  cfblk1 : Inport
  Action Port : ActionPort  ActionPortLabel=if(u1 >= 0)
  cfblk3 : simulink/Discrete/Transfer Fcn Lead or Lag  PoleZ=0.95  ZeroZ=0.75  ICPrevOutput=0.0  ICPrevInput=0.0  DoSatur=off
      settings: SourceProductBaseCode=SL
  cfblk4 : DiscreteFilter
  cfblk5 : Constant  Value=[533791565.201880]  SampleTime=1
  cfblk2 : Outport
  wires:
  cfblk1/1 -> cfblk2/1
  cfblk5/1 -> cfblk3/1
  cfblk3/1 -> cfblk4/1

== system sampleModel248/cfblk88 ==
  cfblk1 : Inport
  Action Port : ActionPort  ActionPortLabel=else
  cfblk3 : UnitDelay  SampleTime=-1  HasFrameUpgradeWarning=on
  cfblk2 : Outport
  wires:
  cfblk1/1 -> cfblk3/1
  cfblk3/1 -> cfblk2/1

== system sampleModel248/cfblk89 ==
  cfblk1 : Inport
  Action Port : ActionPort  ActionPortLabel=if(u1 >= 0)
  cfblk3 : DiscreteZeroPole  Poles=[0 0.5]  Gain=1  SampleTime=-1
  cfblk2 : Outport
  wires:
  cfblk1/1 -> cfblk3/1
  cfblk3/1 -> cfblk2/1

== system sampleModel248/cfblk90 ==
  cfblk1 : Inport
  cfblk3 : Inport  Port=2
  Action Port : ActionPort  ActionPortLabel=else
  cfblk2 : Outport
  wires:
  cfblk3/1 -> cfblk2/1

== system sampleModel248/cfblk91 ==
  cfblk1 : Inport
  Action Port : ActionPort  ActionPortLabel=if(u1 >= 0)
  cfblk3 : Squeeze
  cfblk2 : Outport
  wires:
  cfblk1/1 -> cfblk3/1
  cfblk3/1 -> cfblk2/1

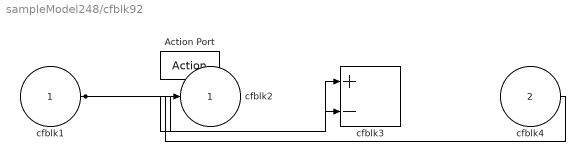
== system sampleModel248/cfblk92 ==
  cfblk1 : Inport
  cfblk4 : Inport  Port=2
  Action Port : ActionPort  ActionPortLabel=else
  cfblk3 : Sum  Inputs=+-
  cfblk2 : Outport
  wires:
  cfblk1/1 -> cfblk3/1, cfblk3/2
  cfblk4/1 -> cfblk2/1

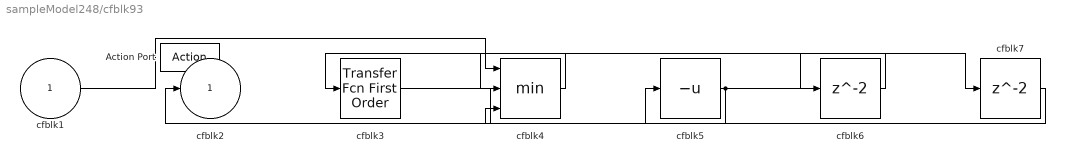
== system sampleModel248/cfblk93 ==
  cfblk1 : Inport
  Action Port : ActionPort  ActionPortLabel=if(u1 >= 0)
  cfblk3 : simulink/Discrete/Transfer Fcn First Order  PoleZ=0.95  ICPrevOutput=0.0  DoSatur=off
  cfblk4 : MinMax  Inputs=3
  cfblk5 : UnaryMinus
  cfblk6 : Delay
  cfblk7 : Delay
  cfblk2 : Outport
  wires:
  cfblk5/1 -> cfblk2/1, cfblk6/1, cfblk7/1
  cfblk1/1 -> cfblk4/1
  cfblk4/1 -> cfblk3/1
  cfblk3/1 -> cfblk5/1
  cfblk6/1 -> cfblk4/2
  cfblk7/1 -> cfblk4/3

== system sampleModel248/cfblk94 ==
  cfblk1 : Inport
  Action Port : ActionPort  ActionPortLabel=else
  cfblk3 : simulink/Discrete/Tapped Delay  vinit=0.0  samptime=-1  NumDelays=1  DelayOrder=Oldest  includeCurrent=off
  cfblk2 : Outport
  wires:
  cfblk3/1 -> cfblk2/1
  cfblk1/1 -> cfblk3/1
